simulink model "controladores1"  (R2018b)
settings: Solver=ode4  StartTime=0.0  StopTime=10  FixedStep=0.0001  RelTol=1e-3
undefined symbols (not defined in the file): Gc1p, Gcdbn, kp, kv, Tm
settings Model: Creator=Vflrz17  LastModifiedBy=a4lfr
settings SFSimCC: SimUseLocalCustomCode=off
settings RTWCC: RTWUseLocalCustomCode=off

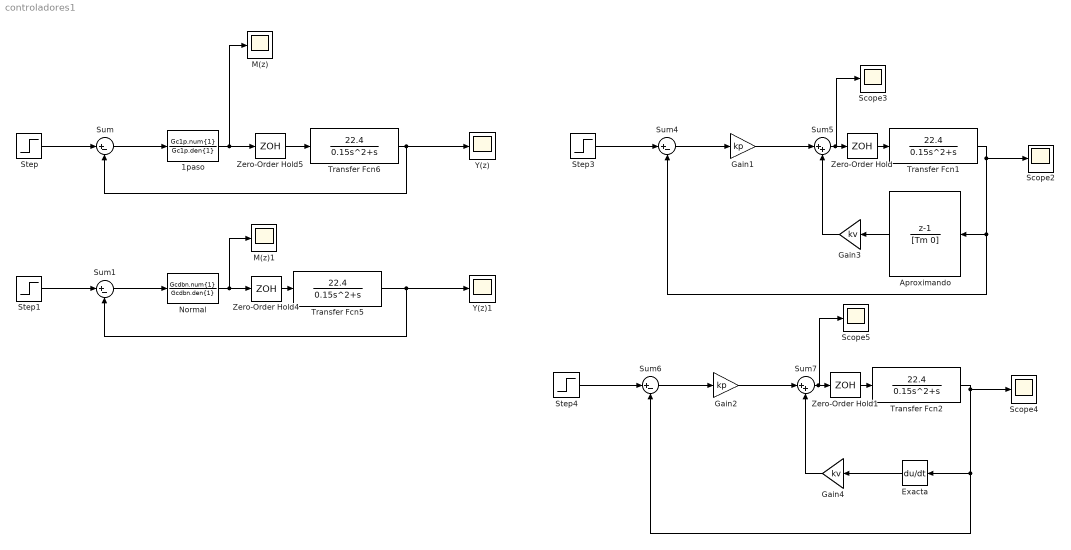
== system controladores1 ==
  1paso : DiscreteTransferFcn  Numerator=Gc1p.num{1}  Denominator=Gc1p.den{1}
  Aproximando : DiscreteTransferFcn  Numerator=[1 -1]  Denominator=[Tm 0]  SampleTime=0.002
  Exacta : Derivative
  Gain1 : Gain  Gain=kp
  Gain2 : Gain  Gain=kp
  Gain3 : Gain  Gain=kv
  Gain4 : Gain  Gain=kv
  M(z) : Scope
  M(z)1 : Scope
  Normal : DiscreteTransferFcn  Numerator=Gcdbn.num{1}  Denominator=Gcdbn.den{1}
  Scope{2..5} (4 alike) : Scope
  Step : Step  SampleTime=0
  Step1 : Step  SampleTime=0
  Step3 : Step  Time=0  SampleTime=0
  Step4 : Step  Time=0  SampleTime=0
  Sum{,1,4,6} (4 alike) : Sum  Inputs=|+-
  Sum5 : Sum  Inputs=|++
  Sum7 : Sum  Inputs=|++
  Transfer Fcn{1..2,5..6} (4 alike) : TransferFcn  Numerator=[22.4]  Denominator=[0.15 1 0]
  Y(z) : Scope
  Y(z)1 : Scope
  Zero-Order Hold{,1,4..5} (4 alike) : ZeroOrderHold  SampleTime=0.03
  wires:
  1paso/1 -> Zero-Order Hold5/1, M(z)/1
  Sum/1 -> 1paso/1
  Transfer Fcn6/1 -> Sum/2, Y(z)/1
  Step/1 -> Sum/1
  Normal/1 -> Zero-Order Hold4/1, M(z)1/1
  Sum1/1 -> Normal/1
  Step1/1 -> Sum1/1
  Transfer Fcn5/1 -> Sum1/2, Y(z)1/1
  Step3/1 -> Sum4/1
  Transfer Fcn1/1 -> Sum4/2, Aproximando/1, Scope2/1
  Sum4/1 -> Gain1/1
  Gain3/1 -> Sum5/2
  Aproximando/1 -> Gain3/1
  Gain1/1 -> Sum5/1
  Sum5/1 -> Scope3/1, Zero-Order Hold/1
  Zero-Order Hold/1 -> Transfer Fcn1/1
  Zero-Order Hold1/1 -> Transfer Fcn2/1
  Gain2/1 -> Sum7/1
  Gain4/1 -> Sum7/2
  Exacta/1 -> Gain4/1
  Sum6/1 -> Gain2/1
  Step4/1 -> Sum6/1
  Transfer Fcn2/1 -> Exacta/1, Sum6/2, Scope4/1
  Zero-Order Hold4/1 -> Transfer Fcn5/1
  Zero-Order Hold5/1 -> Transfer Fcn6/1
  Sum7/1 -> Scope5/1, Zero-Order Hold1/1
